simulink model "Fig412"  (R2014b)
settings: Solver=FixedStepDiscrete  StartTime=0.0  StopTime=0.65536  RelTol=1e-3
libraries: dspsigops x1
settings Model: Creator=Dennis Silage  LastModifiedBy=Silage
settings DataIOCC: SignalLoggingSaveFormat=ModelDataLogs
settings OptimizationCC: ExpressionDepthLimit=2147483647  InitFltsAndDblsToZero=on
settings DebuggingCC: UnderspecifiedInitializationDetection=Classic  MergeDetectMultiDrivingBlocksExec=none  FcnCallInpInsideContextMsg=UseLocalSettings  StateNameClashWarn=warning
settings GRTTargetCC: CombineOutputUpdateFcns=off  GRTInterface=on

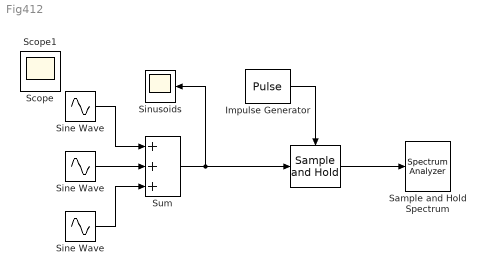
== system Fig412 ==
  "   " : dspsigops/Sample and Hold  trig=Rising edge  initCond=0  latchinput=off
  " Sine Wave " : Sin  Amplitude=0.2  Frequency=5000*pi  SampleTime=1.25e-6
  Impulse Generator : DiscretePulseGenerator  Period=229  SampleTime=1.25e-6
  Sample and Hold Spectrum : SpectrumAnalyzer
  Sine Wave : Sin  Frequency=1000*pi  SampleTime=1.25e-6
  "Sine Wave " : Sin  Amplitude=0.5  Frequency=3000*pi  SampleTime=1.25e-6
  Sinusoids : Scope
      settings: YMin=-1.5  YMax=1.5
  Sum : Sum  Inputs=+++
  Scope : Scope
      settings: MaxDataPoints=7500  SampleTime=-1
  Scope1 : Scope
      settings: MaxDataPoints=7500  SampleTime=-1
  wires:
  "Sine Wave "/1 -> Sum/2
  " Sine Wave "/1 -> Sum/3
  Sine Wave/1 -> Sum/1
  Sum/1 -> "   "/1, Sinusoids/1
  Impulse Generator/1 -> "   "/Trigger
  "   "/1 -> Sample and Hold Spectrum/1
